simulink model "Nelinearni_realni"  (R2023b)
settings: Solver=ode23t  StartTime=0.0  StopTime=stepp.sim_time  RelTol=1e-3
undefined symbols (not defined in the file): Bat, boost, ccm_op, Ci, dcm_op_cv, G_ccm, Gp_dcm_cv, pv_data, pv_eq, pv_in, sim_op, stepp
libraries: spsSeriesRLCBranchLib x5, spsCurrentMeasurementLib x4, spsVoltageMeasurementLib x3, spsControlledVoltageSourceLib x2, spsControlledCurrentSourceLib x1, spsDiodeLib x1, spsIdealSwitchLib x1, sps_lib x1
settings Model: Creator=teo  LastModifiedBy=teo

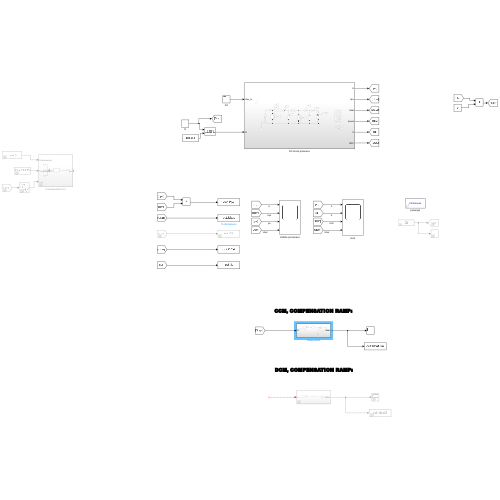
[thumbnail: Simulink's stored preview of the top-level diagram]
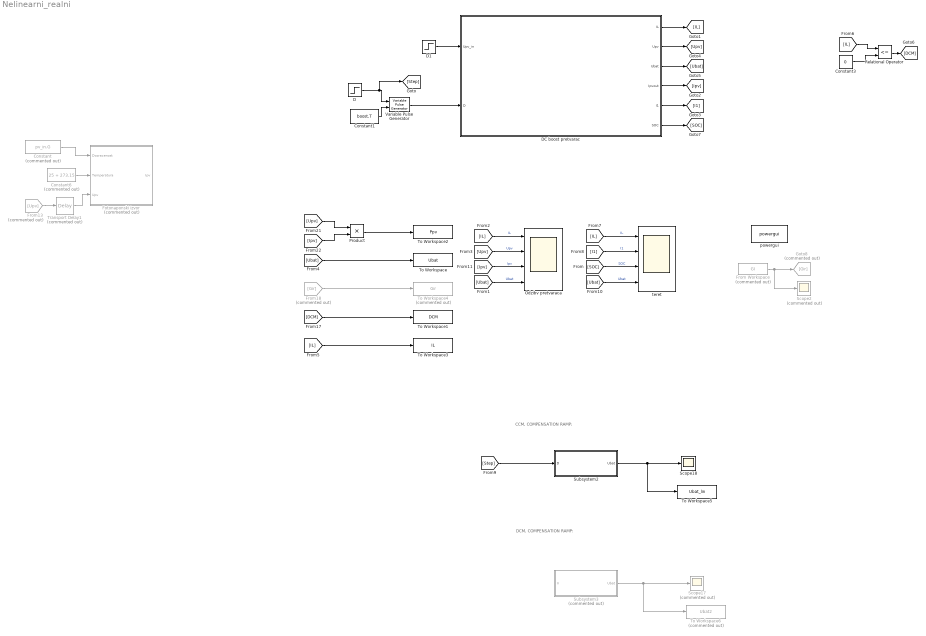
== system Nelinearni_realni ==
  note: DCM, COMPENSATION RAMP:
  note: CCM, COMPENSATION RAMP:
  Constant : Constant  Commented=on  Value=pv_in.G
  Constant1 : Constant  Value=boost.T
  Constant3 : Constant  Value=0
  Constant6 : Constant  Commented=on  Value=25 + 273.15
  D : Step  Time=stepp.step_time  Before=stepp.D1  After=stepp.D2  SampleTime=0
  D1 : Step  Time=stepp.step_time  Before=stepp.Upv1  After=stepp.Upv2  SampleTime=0
  DC boost pretvarac : Subsystem
  Fotonaponski izvor : Subsystem  Commented=on
  From Workspace : FromWorkspace  Commented=on  VariableName=GI
  From13 : From  Commented=on  GotoTag=Upv
  From18 : From  Commented=on  GotoTag=Gir
  Goto8 : Goto  Commented=on  GotoTag=Gir
  Odzibv pretvaraca : Scope  NumInputPorts=4
  Product : Product
  Relational Operator : RelationalOperator  Operator=<=  OutDataTypeStr=boolean  RndMeth=Simplest  InputSameDT=off
  Scope17 : Scope  Commented=on
  Scope18 : Scope
  Scope2 : Scope  Commented=on
  Subsystem2 : Subsystem
  Subsystem3 : Subsystem  Commented=on
  To Workspace : ToWorkspace  VariableName=Ubat  SaveFormat=Timeseries  SampleTime=-1
  To Workspace1 : ToWorkspace  VariableName=DCM  SaveFormat=Timeseries  SampleTime=-1
  To Workspace2 : ToWorkspace  VariableName=Ppv  SaveFormat=Timeseries  SampleTime=-1
  To Workspace3 : ToWorkspace  VariableName=IL  SaveFormat=Timeseries  SampleTime=-1
  To Workspace4 : ToWorkspace  Commented=on  VariableName=Gir  SaveFormat=Timeseries  SampleTime=-1
  To Workspace5 : ToWorkspace  VariableName=Ubat_lin  SaveFormat=Timeseries  SampleTime=-1
  To Workspace6 : ToWorkspace  Commented=on  VariableName=Ubat2  SaveFormat=Timeseries  SampleTime=1e-6
  Transport Delay1 : TransportDelay  Commented=on  DelayTime=0.0001  BufferSize=4024
  Variable Pulse Generator : VariablePulseGenerator  SampleTime=0.1
  powergui : sps_lib/powergui  Priority=1  SimulationMode=Continuous  SampleTime=50e-6  frequency=60  Iterations=50  frequencyindice=0  Pbase=100e6  ErrMax=1e-4  UnitsV=kV  UnitsW=MW  buscounter=0  FunctionMessages=off  echomessages=off  EnableUseOfTLC=off  CurrentSourceSwitches=off  DisableSnubberDevices=off  DisableRonSwitches=off  DisableVfSwitches=off  DisplayEquations=off  AutomaticDiscreteSolvers=off  SolverType=Tustin/Backward Euler (TBE)  Interpol=off  ExternalGateDelay=off  methode=off  Ts=100  x0status=blocks  SPID=on  SwTol=0  HookPort=off  NonlinearTolerance=1e-4  nMaxIteration=100  ContinueOnMaxIteration=off  RestoreLinks=warning  ResistiveCurrentMeasurement=off  Frange=[0:2:500]  Ylog=off  Xlog=on  ShowGrid=off  save=off  variable=ZData  structure=0  ZoomFFT=off  StartTime=0.0  cycles=1  DisplayStyle=1  fundamental=60  FreqAxis=off  MaxFrequency=1000  frequencyindicesteady=1  RmsSteady=1  display=off
  teret : Scope  NumInputPorts=4
  wires:
  [IL] -> Relational Operator/1
  Relational Operator/1 -> [DCM]
  Constant3/1 -> Relational Operator/2
  Constant6/1 -> Fotonaponski izvor/2(Temperatura)
  Transport Delay1/1 -> Fotonaponski izvor/3(Upv)
  DC boost pretvarac/6(SOC) -> [SOC]
  DC boost pretvarac/1(IL) -> [IL]
  DC boost pretvarac/5(I1) -> [I1]
  DC boost pretvarac/3(Ubat) -> [Ubat]
  DC boost pretvarac/4(Ipvout) -> [Ipv]
  DC boost pretvarac/2(Upv) -> [Upv]
  From13/1 -> Transport Delay1/1
  [Upv] -> Product/1
  [Ubat] -> teret/4  "Ubat"
  [Ipv] -> Product/2
  [IL] -> Odzibv pretvaraca/1  "IL"
  From Workspace/1 -> Scope2/1, Goto8/1
  Product/1 -> To Workspace2/1
  [SOC] -> teret/3  "SOC"
  [Ipv] -> Odzibv pretvaraca/3  "Ipv"
  [Upv] -> Odzibv pretvaraca/2  "Upv"
  [DCM] -> To Workspace1/1
  From18/1 -> To Workspace4/1
  [Ubat] -> To Workspace/1
  [I1] -> teret/2  "I1"
  [Ubat] -> Odzibv pretvaraca/4  "Ubat"
  [IL] -> teret/1  "IL"
  Constant/1 -> Fotonaponski izvor/1(Dozracenost)
  Constant1/1 -> Variable Pulse Generator/2
  D/1 -> [Step], Variable Pulse Generator/1
  Variable Pulse Generator/1 -> DC boost pretvarac/2(D)
  [IL] -> To Workspace3/1
  Subsystem3/1(Ubat) -> To Workspace6/1, Scope17/1
  [Step] -> Subsystem2/1(D)
  ? -> Subsystem3/1(Ir)
  Subsystem2/1(Ubat) -> Scope18/1, To Workspace5/1
  D1/1 -> DC boost pretvarac/1(Upv_in)

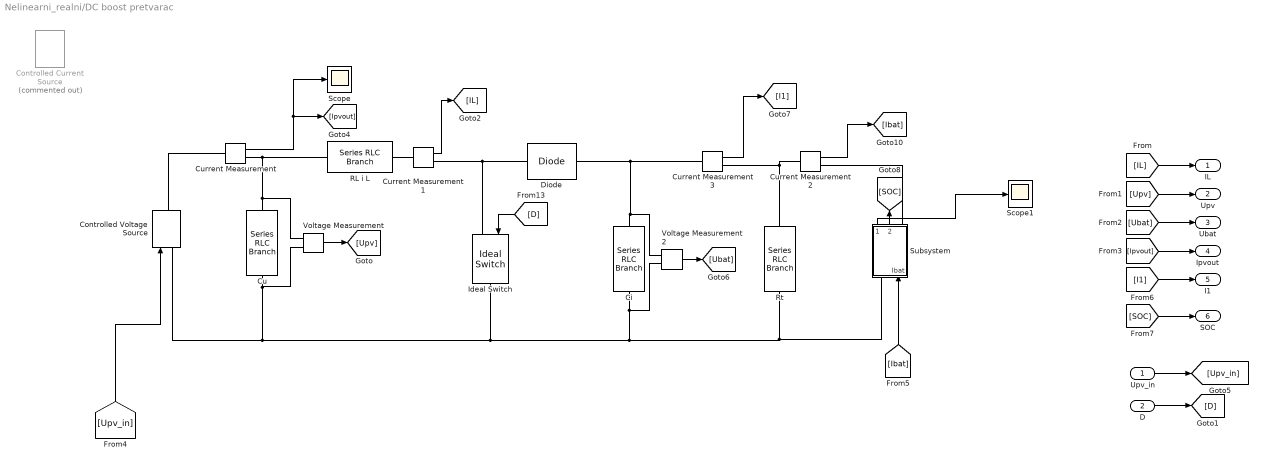
== system Nelinearni_realni/DC boost pretvarac ==
  Upv_in : Inport
  D : Inport  Port=2
  Ci : spsSeriesRLCBranchLib/Series RLC Branch  LConnTagsString=__new0  RConnTagsString=__new0  BranchType=C  Resistance=0.001  Inductance=1e-3  SetiL0=off  InitialCurrent=0  Capacitance=boost.Ci  Setx0=on  InitialVoltage=sim_op.Ubat0  Measurements=None
  Controlled Current Source : spsControlledCurrentSourceLib/Controlled Current Source  Commented=on  Initialize=on  Source_Type=AC  Amplitude=0  Phase=0  Frequency=0  Measurements=None
  Controlled Voltage Source : spsControlledVoltageSourceLib/Controlled Voltage Source  Initialize=on  Source_Type=DC  Amplitude=sim_op.Upv0  Phase=0  Frequency=0  Measurements=None
  Cu : spsSeriesRLCBranchLib/Series RLC Branch  LConnTagsString=__new0  RConnTagsString=__new0  BranchType=RC  Resistance=0.001  Inductance=1e-3  SetiL0=off  InitialCurrent=0  Capacitance=boost.Cu  Setx0=on  InitialVoltage=sim_op.Upv0  Measurements=None
  Current Measurement{,1..3} (4 alike) : spsCurrentMeasurementLib/Current Measurement  PhasorSimulation=off  OutputType=Complex  PSBequivalent=0
  Diode : spsDiodeLib/Diode  Ron=0  Lon=0  Vf=0  IC=0  UseSnubber=0  Rs=0  Cs=0  Measurements=off
  Ideal Switch : spsIdealSwitchLib/Ideal Switch  Ron=0  Lon=0  IC=0  Rs=0  Cs=0  Measurements=off
  RL i L : spsSeriesRLCBranchLib/Series RLC Branch  LConnTagsString=__new0  RConnTagsString=__new0  BranchType=RL  Resistance=boost.RL  Inductance=boost.L  SetiL0=off  InitialCurrent=stepp.ir01  Capacitance=1e-6  Setx0=off  InitialVoltage=0  Measurements=None
  Rt : spsSeriesRLCBranchLib/Series RLC Branch  LConnTagsString=__new0  RConnTagsString=__new0  BranchType=R  Resistance=boost.Rt  Inductance=1e-3  SetiL0=off  InitialCurrent=0  Capacitance=Ci  Setx0=off  InitialVoltage=0  Measurements=None
  Scope : Scope
  Scope1 : Scope
  Subsystem : Subsystem
      settings: PortSchema="{\"entries\":[{\"content\":{\"sides\":[{\"content\":{\"connectorIds\":[\"LConn1\",\"In1\"]},\"type\":\"ConnectorPlacement.EquallySpacedRectSide\",\"uuid\":\"36a151cb-ade8-4d77-9227-5d94720a867f\"},{\"content\":{\"connectorIds\":[\"Out1\",\"Out2\",\"RConn1\"],\"side\":\"RIGHT\"},\"type\":\"ConnectorPlacement.EquallySpacedRectSide\",\"uuid\":\"e273b59b-5ac5-431a-9422-aa1eb85d6b42\"},{\"content\":{\"side\":\"TOP\"},\"type\":\"ConnectorPlacement.EquallySpacedRectSide\",\"uuid\":\"963da400-5a20-4c48-ad4c-e087b1b0be12\"}]},\"type\":\"ConnectorPlacement.EquallySpacedConnector\",\"uuid\":\"3f6c7281-abab-4595-a869-b172f12b4791\"}],\"packageUris\":[\"http://schema.mathworks.com/mf0/Connector/R2020b\"],\"version\":\"1.0\"}"
  Voltage Measurement : spsVoltageMeasurementLib/Voltage Measurement  PhasorSimulation=off  OutputType=Complex  PSBequivalent=0
  Voltage Measurement2 : spsVoltageMeasurementLib/Voltage Measurement  PhasorSimulation=off  OutputType=Complex  PSBequivalent=0
  IL : Outport
  Upv : Outport  Port=2
  Ubat : Outport  Port=3
  Ipvout : Outport  Port=4
  I1 : Outport  Port=5
  SOC : Outport  Port=6
  wires:
  Current Measurement1/1 -> [IL]
  Voltage Measurement/1 -> [Upv]
  [D] -> Ideal Switch/1
  D/1 -> [D]
  Upv_in/1 -> [Upv_in]
  [IL] -> IL/1
  [Upv] -> Upv/1
  [Ubat] -> Ubat/1
  Current Measurement/1 -> Scope/1, [Ipvout]
  [Ipvout] -> Ipvout/1
  [I1] -> I1/1
  Voltage Measurement2/1 -> [Ubat]
  Current Measurement2/1 -> [Ibat]
  [Ibat] -> Subsystem/1(Ibat)
  Current Measurement3/1 -> [I1]
  [SOC] -> SOC/1
  Subsystem/2(SOC) -> [SOC]
  Subsystem/1(Uoc) -> Scope1/1
  [Upv_in] -> Controlled Voltage Source/1
  connections:
  Current Measurement/RConn1 -- Voltage Measurement/LConn1 -- Cu/LConn1 -- RL i L/LConn1
  RL i L/RConn1 -- Current Measurement1/LConn1
  Diode/LConn1 -- Ideal Switch/LConn1 -- Current Measurement1/RConn1
  Ci/RConn1 -- Voltage Measurement2/LConn2 -- Subsystem/LConn1 -- Rt/RConn1 -- Controlled Voltage Source/LConn1 -- Voltage Measurement/LConn2 -- Cu/RConn1 -- Ideal Switch/RConn1
  Voltage Measurement2/LConn1 -- Current Measurement3/LConn1 -- Diode/RConn1 -- Ci/LConn1
  Subsystem/RConn1 -- Current Measurement2/RConn1
  Rt/LConn1 -- Current Measurement3/RConn1 -- Current Measurement2/LConn1
  Controlled Voltage Source/RConn1 -- Current Measurement/LConn1

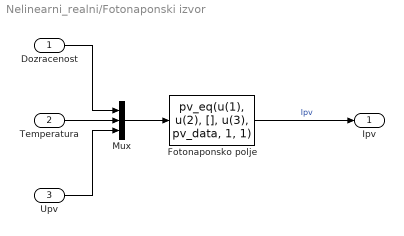
== system Nelinearni_realni/Fotonaponski izvor ==
  Dozracenost : Inport
  Temperatura : Inport  Port=2
  Upv : Inport  Port=3
  Fotonaponsko polje : MATLABFcn  MATLABFcn=pv_eq(u(1), u(2), [], u(3), pv_data, 1, 1)  OutputDimensions=1
  Mux : Mux  Inputs=3
  Ipv : Outport
  wires:
  Fotonaponsko polje/1 -> Ipv/1  "Ipv"
  Mux/1 -> Fotonaponsko polje/1
  Dozracenost/1 -> Mux/1
  Temperatura/1 -> Mux/2
  Upv/1 -> Mux/3

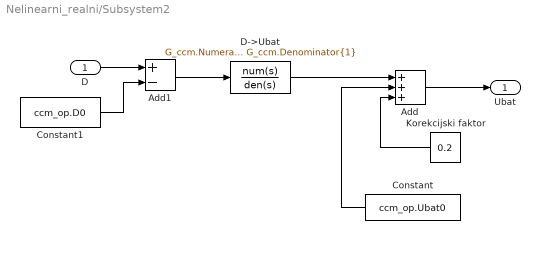
== system Nelinearni_realni/Subsystem2 ==
  D : Inport
  Add : Sum  Inputs=+++
  Add1 : Sum  Inputs=+-
  Constant : Constant  Value=ccm_op.Ubat0
  Constant1 : Constant  Value=ccm_op.D0
  D->Ubat : TransferFcn  Numerator=G_ccm.Numerator{1}  Denominator=G_ccm.Denominator{1}
  Korekcijski faktor : Constant  Value=0.2
  Ubat : Outport
  wires:
  D/1 -> Add1/1
  Constant1/1 -> Add1/2
  Add1/1 -> D->Ubat/1
  Add/1 -> Ubat/1
  Constant/1 -> Add/2
  D->Ubat/1 -> Add/1
  Korekcijski faktor/1 -> Add/3

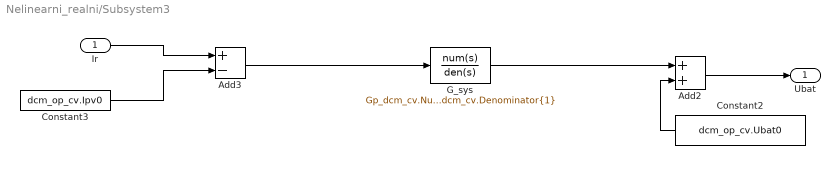
== system Nelinearni_realni/Subsystem3 ==
  Ir : Inport
  Add2 : Sum
  Add3 : Sum  Inputs=+-
  Constant2 : Constant  Value=dcm_op_cv.Ubat0
  Constant3 : Constant  Value=dcm_op_cv.Ipv0
  G_sys : TransferFcn  Numerator=Gp_dcm_cv.Numerator{1}  Denominator=Gp_dcm_cv.Denominator{1}
  Ubat : Outport
  wires:
  Constant3/1 -> Add3/2
  Add3/1 -> G_sys/1
  G_sys/1 -> Add2/1
  Constant2/1 -> Add2/2
  Ir/1 -> Add3/1
  Add2/1 -> Ubat/1

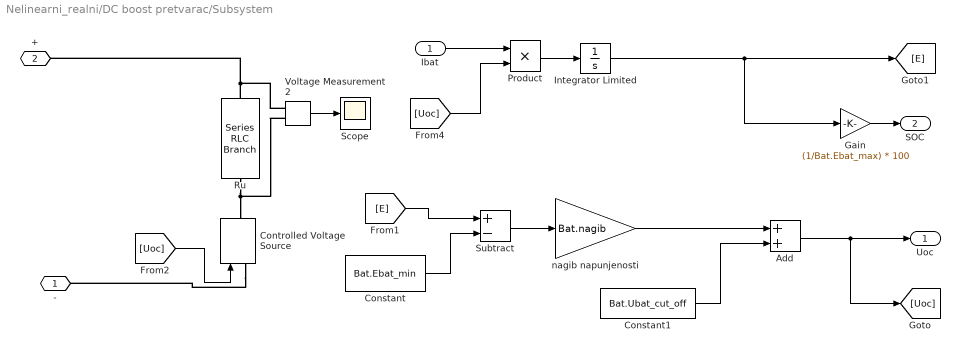
== system Nelinearni_realni/DC boost pretvarac/Subsystem ==
  Ibat : Inport
  Add : Sum
  Constant : Constant  Value=Bat.Ebat_min
  Constant1 : Constant  Value=Bat.Ubat_cut_off
  Controlled Voltage Source : spsControlledVoltageSourceLib/Controlled Voltage Source  Initialize=on  Source_Type=DC  Amplitude=sim_op.Ubat0  Phase=0  Frequency=0  Measurements=None
  Gain : Gain  Gain=(1/Bat.Ebat_max) * 100
  Integrator Limited : Integrator  InitialCondition=sim_op.E0  LimitOutput=on  UpperSaturationLimit=Bat.Ebat_max  LowerSaturationLimit=Bat.Ebat_min
  Product : Product
  Ru : spsSeriesRLCBranchLib/Series RLC Branch  LConnTagsString=__new0  RConnTagsString=__new0  BranchType=R  Resistance=boost.Ru  Inductance=1e-3  SetiL0=off  InitialCurrent=0  Capacitance=Ci  Setx0=off  InitialVoltage=0  Measurements=None
  Scope : Scope
  Subtract : Sum  Inputs=+-
  Voltage Measurement2 : spsVoltageMeasurementLib/Voltage Measurement  PhasorSimulation=off  OutputType=Complex  PSBequivalent=0
  nagib napunjenosti : Gain  Gain=Bat.nagib
  - : PMIOPort  Side=Left
  + : PMIOPort  Port=2  Side=Right
  Uoc : Outport
  SOC : Outport  Port=2
  wires:
  Subtract/1 -> nagib napunjenosti/1
  Constant/1 -> Subtract/2
  nagib napunjenosti/1 -> Add/1
  Constant1/1 -> Add/2
  Integrator Limited/1 -> Gain/1, [E]
  [Uoc] -> Product/2
  Product/1 -> Integrator Limited/1
  Ibat/1 -> Product/1
  [E] -> Subtract/1
  [Uoc] -> Controlled Voltage Source/1
  Gain/1 -> SOC/1
  Add/1 -> Uoc/1, [Uoc]
  Voltage Measurement2/1 -> Scope/1
  connections:
  Controlled Voltage Source/LConn1 -- -/RConn1
  Ru/RConn1 -- Voltage Measurement2/LConn2 -- Controlled Voltage Source/RConn1
  Ru/LConn1 -- Voltage Measurement2/LConn1 -- +/RConn1
